simulink model "Project8Simulink"  (R2020a)
settings: Solver=VariableStepAuto  StartTime=0.0  StopTime=Sim_time  RelTol=1e-3
values from neighbouring files (symbols this model uses):
  b = 10    [Project8.m]    (also in Project9.m)
  kd = 100    [Project8.m]    (also in Project9.m)
  ki = 50    [Project8.m]    (also in Project9.m)
  kp = 500    [Project8.m]    (also in Project9.m)
  m = 1    [Project8.m]    (also in Project9.m)
  Sim_step = 1    [Project8.m]    (also in Project9.m)
settings Model: Creator=cresp  LastModifiedBy=cresp

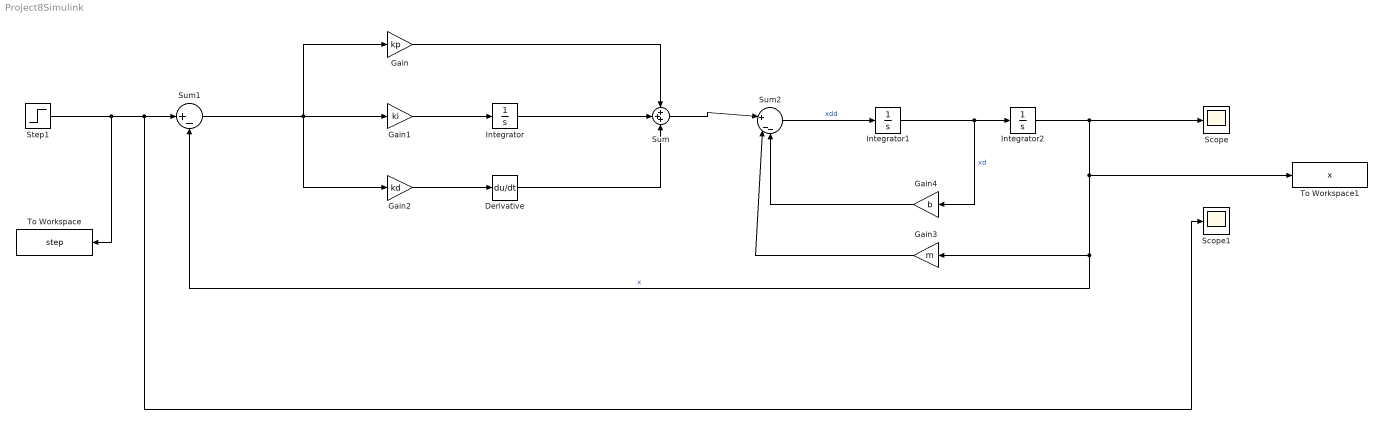
== system Project8Simulink ==
  Derivative : Derivative
  Gain : Gain  Gain=kp
  Gain1 : Gain  Gain=ki
  Gain2 : Gain  Gain=kd
  Gain3 : Gain  Gain=m
  Gain4 : Gain  Gain=b
  Integrator : Integrator
  Integrator1 : Integrator
  Integrator2 : Integrator
  Scope : Scope
  Scope1 : Scope
  Step1 : Step  Time=Sim_step  SampleTime=0
  Sum : Sum  Inputs=+++
  Sum1 : Sum  Inputs=|+-
  Sum2 : Sum  Inputs=||+|--
  To Workspace : ToWorkspace  VariableName=step  SaveFormat=Timeseries  SampleTime=-1
  To Workspace1 : ToWorkspace  VariableName=x  SaveFormat=Timeseries  SampleTime=-1
  wires:
  Gain/1 -> Sum/1
  Integrator/1 -> Sum/2
  Gain1/1 -> Integrator/1
  Gain2/1 -> Derivative/1
  Sum1/1 -> Gain/1, Gain1/1, Gain2/1
  Derivative/1 -> Sum/3
  Integrator1/1 -> Gain4/1, Integrator2/1  "xd"
  Sum/1 -> Sum2/1
  Step1/1 -> To Workspace/1, Scope1/1, Sum1/1
  Sum2/1 -> Integrator1/1  "xdd"
  Integrator2/1 -> Scope/1, Gain3/1, Sum1/2, To Workspace1/1  "x"
  Gain3/1 -> Sum2/2
  Gain4/1 -> Sum2/3
